simulink model "test"  (R2026a)
settings: Solver=VariableStepAuto
libraries: sl_discontinuities x1
settings Model: Creator=chris  LastModifiedBy=chris

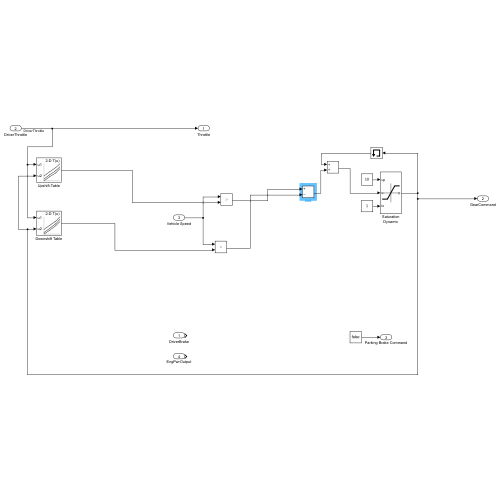
[thumbnail: Simulink's stored preview of the top-level diagram]
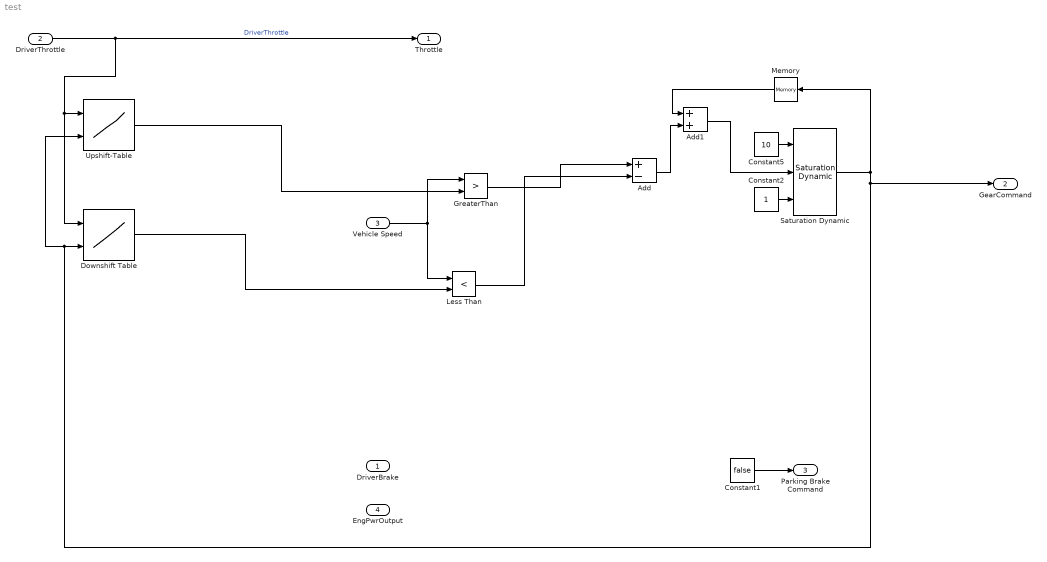
== system test ==
  DriverBrake : Inport  OutDataTypeStr=double  PortDimensions=1
  DriverThrottle : Inport  Port=2  OutDataTypeStr=double  PortDimensions=1
  Vehicle Speed : Inport  Port=3  OutDataTypeStr=double  PortDimensions=1
  EngPwrOutput : Inport  Port=4
  Add : Sum  Inputs=+-  SaturateOnIntegerOverflow=on
  Add1 : Sum  SaturateOnIntegerOverflow=on
  Constant1 : Constant  Value=false
  Constant2 : Constant
  Constant5 : Constant  Value=10
  Downshift Table : Lookup_n-D  BreakpointsForDimension1=[0.2 0.5 0.8 1.0]  BreakpointsForDimension2=[1:3]  Table=[15 32 50 68; 22 40 58 78; 35 52 70 88]'  InternalRulePriority=Speed  RndMeth=Simplest
      settings: InputPortMap=u0,u1
  GreaterThan : RelationalOperator  Operator=>  OutDataTypeStr=boolean  RndMeth=Simplest  InputSameDT=off
  Less Than : RelationalOperator  Operator=<  OutDataTypeStr=boolean  RndMeth=Simplest  InputSameDT=off
  Memory : Memory  InheritSampleTime=on
  Saturation Dynamic : sl_discontinuities/Saturation Dynamic  OutMin=[]  OutMax=[]  OutDataTypeStr=Inherit: Same as second input  OutDataType=fixdt(1, 16)  OutScaling=2^-10  DoSatur=off
      settings: LibrarySourceBlock=|
      | simulink/Discontinuities/Saturation
      | Dynamic
  Upshift-Table : Lookup_n-D  BreakpointsForDimension1=[0.2 0.5 0.8 1.0]  BreakpointsForDimension2=[1:3]  Table=[25 45 65 85; 35 55 75 95; 50 70 90 110]'  InternalRulePriority=Speed  RndMeth=Simplest
      settings: InputPortMap=u0,u1
  Throttle : Outport  OutDataTypeStr=double  PortDimensions=1
  GearCommand : Outport  Port=2  OutDataTypeStr=double  PortDimensions=1
  Parking Brake Command : Outport  Port=3  OutDataTypeStr=boolean  PortDimensions=1
  wires:
  GreaterThan/1 -> Add/1
  Less Than/1 -> Add/2
  Add/1 -> Add1/2
  Add1/1 -> Saturation Dynamic/2
  Memory/1 -> Add1/1
  Constant2/1 -> Saturation Dynamic/3
  Vehicle Speed/1 -> Less Than/1, GreaterThan/1
  Saturation Dynamic/1 -> GearCommand/1, Upshift-Table/2, Downshift Table/2, Memory/1
  Constant1/1 -> Parking Brake Command/1
  DriverThrottle/1 -> Downshift Table/1, Upshift-Table/1, Throttle/1  "DriverThrottle"
  Constant5/1 -> Saturation Dynamic/1
  Upshift-Table/1 -> GreaterThan/2
  Downshift Table/1 -> Less Than/2
